simulink model "SF5_5_6_na0013"  (R2016b)
settings: Solver=FixedStepDiscrete  StartTime=0.0  StopTime=10.0  RelTol=1e-3  EnableMultiTasking=on
settings Model: Creator=amyyang  LastModifiedBy=amyyang
settings DataIOCC: LimitDataPoints=on
settings OptimizationCC: DefaultParameterBehavior=Inlined  LifeSpan=1
settings DebuggingCC: AllowSymbolicDim=off  SFUnexpectedBacktrackingDiag=warning  SFNoUnconditionalDefaultTransitionDiag=warning  SFExecutionAtInitializationDiag=none
settings ModelReferenceCC: PropagateSignalLabelsOutOfModel=off
settings RTWCC: SystemTargetFile=ert.tlc  GenCodeOnly=on  TemplateMakefile=ert_default_tmf  Description=Embedded Coder  GenerateReport=on  IncludeHyperlinkInReport=on  LaunchReport=on  GenerateTraceInfo=on  GenerateTraceReport=on  GenerateTraceReportSl=on  GenerateTraceReportSf=on  GenerateTraceReportEml=on
settings CodeAppCC: IgnoreCustomStorageClasses=off
settings ERTTargetCC: GenerateSampleERTMain=on  InlinedParameterPlacement=NonHierarchical  ERTCustomFileTemplate=example_file_process.tlc  ConvertIfToSwitch=off  SuppressUnreachableDefaultCases=off
settings ConfigComp: CovMetricSettings=dw  CovHtmlReporting=on  CovSaveCumulativeToWorkspaceVar=on  CovSaveSingleToWorkspaceVar=on  CovExternalEMLEnable=off

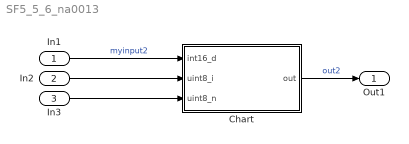
== system SF5_5_6_na0013 ==
  In1 : Inport
  In2 : Inport  Port=2
  In3 : Inport  Port=3
  Chart : Stateflow chart  TreatAsAtomicUnit=on
  Out1 : Outport
  wires:
  Chart/1(out) -> Out1/1  "out2"
  In1/1 -> Chart/1(int16_d)  "myinput2"
  In3/1 -> Chart/3(uint8_n)
  In2/1 -> Chart/2(uint8_i)

== stateflow chart SF5_5_6_na0013/Chart ==
  state B [parallel]
    settings: executionOrder=2
    (default) -> (junction 38) : {
        |  diff = double1 - double2;
        | }
    (junction 38) -> (junction 40) [order 1] : [(-LIMIT < diff)&&(diff < LIMIT)]
    (junction 38) -> (junction 41) [order 2]
    (junction 40) -> (junction 42)
    (junction 41) -> (junction 42) [order 1] : [ doubl1 == double2]
    (junction 41) -> (junction 43) [order 2]
    (junction 42) -> (junction 49)
    (junction 49) -> (junction 43)
    (junction 43) -> (junction 52)
  state A [parallel]
    settings: executionOrder=1
    note: [ uint8_i < int16_d]
    (default) -> (junction 13)
    (junction 13) -> (junction 18) [order 1] : [ uint8_i < uint8_n]
    (junction 18) -> (junction 20) : {
        |  out = 1;
        | }
    (junction 13) -> (junction 14) [order 2]
    (junction 14) -> (junction 20) [order 1] : [ int16(uint8_i) < int16_d]
    (junction 20) -> (junction 23) : {
        |  out = 2;
        | }
    (junction 14) -> (junction 16) [order 2]
    (junction 23) -> (junction 16)
    (junction 16) -> (junction 27)
  data: out output; int16_d input int16; uint8_i input uint8; uint8_n input uint8
